simulink model "tricycle_pathstations"  (R2021a)
settings: Solver=VariableStepAuto  StartTime=0.0  StopTime=inf  RelTol=1e-3
InitFcn:
  | i=1
libraries: simulink_extras x3, vehdynlibviscommon x1
settings Model: Creator=EGYPT  LastModifiedBy=Mostafa Ali
settings SolverCC: AlgebraicLoopSolver=TrustRegion
settings DebuggingCC: SFMachineParentedDataDiag=warning

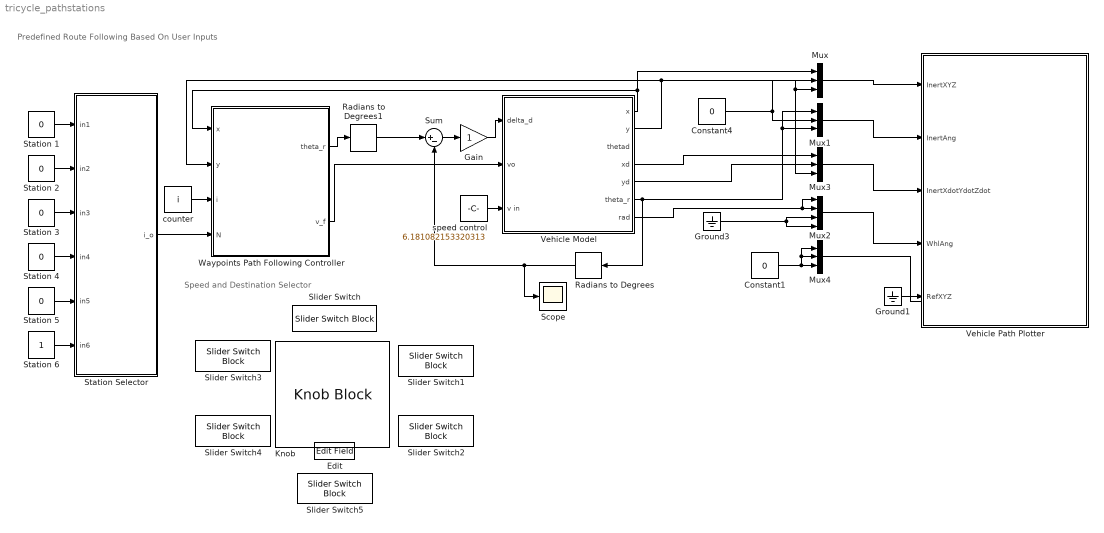
== system tricycle_pathstations ==
  note: Predefined Route Following Based On User Inputs
  note: Speed and Destination Selector
  Constant1 : Constant  Value=0
  Constant4 : Constant  Value=0
  Edit : EditField  LabelPosition=Hide  ShowInitialText=on  Alignment=Center
  Gain : Gain
  Ground1 : Ground
  Ground3 : Ground
  Knob : KnobBlock  ScaleMax=10
  Mux{,1,3..4} (4 alike) : Mux  Inputs=3
  Mux2 : Mux
  Radians to Degrees : simulink_extras/Transformations/Radians to Degrees
  Radians to Degrees1 : simulink_extras/Transformations/Radians to Degrees
  Scope : Scope
  Slider Switch{,1..5} (6 alike) : SliderSwitchBlock
      settings: Values={{'Off', 'On'}, [0 1]}
  Station {1..5} (5 alike) : Constant  Value=0
  Station 6 : Constant
  "Station Selector " : MATLAB Function  TreatAsAtomicUnit=on
  Sum : Sum  Inputs=|+-
  "Vehicle Model " : Subsystem
      mask Display: image('D:\grad 1\matlab\maskKM.JPG'); % Use "Edit Image" on toolstrip to change.
  Vehicle Path Plotter : Subsystem  mask(Vehicle XY Plotter){extRef=on, extStats=off, extTireF=off, a=2, b=2, w=2, figBorder=10, bufferSize=1024, velNorm=5, tireFNorm=1000, pltDT=0.2}
      mask prompts: extRef "Plot path reference, extRef"; extStats "Display speed, RPM and Gear"; extTireF "Display tire forces"; a "Distance to front axle from CG, a [m]:"; b "Distance to rear axle from CG, b [m]:"; w "Track width, w [m]:"; figBorder "Distance to figure borders, figBorder [m]:"; bufferSize "Path buffer sampe size, bufferSize []:"; velNorm "Velocity vector scaling, velNorm [m*s/m]:"; tireFNorm "Tire force vector scaling, tireFNorm [m/N]:"; pltDT "Plot update rate, pltDT [s]:"
      mask help:
      | This block will display a MATLAB figure which indicates the vehicle path, current position and heading velocity.
      | An optional path reference is also provided.
      mask init:
      | block = gcb;
      | if autoblkschecksimstopped(block)
      |     ParamNames = {'extRef';'extStats';'extTireF';'extTireF'};
      |     PortNames = {'RefXYZ';'Stats';'TireFx';'TireFy'};
      |     for idx=1:length(PortNames)
      |         InportOption  = {'built-in/Ground', [PortNames{idx}, ' Ground'];...
      |             'built-in/Inport',PortNames{idx}};
      |         if ~strcmp(get_param(block,ParamNames{idx}),'on')
      |             NewBlkHdl = autoblksreplaceblock(block, InportOption, 1);
      |             set_param(NewBlkHdl, 'ShowName', 'off');
      |         else
      |             autoblksreplaceblock(block, InportOption, 2);
      |         end
      |     end
      |     InportNames = {'InertXYZ';'InertAng';'InertXdotYdotZdot';'WhlAng';'RefXYZ';'Stats';'TireFx';'TireFy'};
      |     FoundNames = get_param(find_system(block, 'LookUnderMasks', 'all', 'SearchDepth', 1, 'FollowLinks', 'on', 'BlockType', 'Inport'), 'Name');
      |     [~,PortI] = intersect(InportNames, FoundNames);
      |     PortI = sort(PortI);
      |     for idx = 1:length(PortI)
      |         set_param([block, '/', InportNames{PortI(idx)}], 'Port', num2str(idx));
      |     end
      | end
      mask TypeOptions a: Vehicle XY Plotter/a
      mask TypeOptions b: Vehicle XY Plotter/b
      mask TypeOptions w: Vehicle XY Plotter/w
      mask TypeOptions figBorder: Vehicle XY Plotter/figBorder
      mask TypeOptions bufferSize: Vehicle XY Plotter/bufferSize
      mask TypeOptions velNorm: Vehicle XY Plotter/velNorm
      mask TypeOptions tireFNorm: Vehicle XY Plotter/tireFNorm
      mask DialogControl Container3 Prompt: Plot and Display Options
  "Waypoints Path Following Controller " : MATLAB Function  TreatAsAtomicUnit=on
  counter : Constant  Value=i
  speed control : Constant  Value=6.181082153320313
  wires:
  Radians to Degrees/1 -> Sum/2, Scope/1
  Mux3/1 -> Vehicle Path Plotter/3(InertXdotYdotZdot)
  "Vehicle Model "/5(yd) -> Mux3/2
  speed control/1 -> "Vehicle Model "/3(v in)
  Radians to Degrees1/1 -> Sum/1
  "Vehicle Model "/1(x) -> Mux/1, "Waypoints Path Following Controller "/1(x)
  Ground3/1 -> Mux2/3, Mux2/4
  "Waypoints Path Following Controller "/1(theta_r) -> Radians to Degrees1/1
  Mux/1 -> Vehicle Path Plotter/1(InertXYZ)
  Sum/1 -> Gain/1
  Mux1/1 -> Vehicle Path Plotter/2(InertAng)
  "Vehicle Model "/2(y) -> Mux/2, "Waypoints Path Following Controller "/2(y)
  "Vehicle Model "/4(xd) -> Mux3/1
  Constant1/1 -> Mux4/1, Mux4/2, Mux4/3
  Mux2/1 -> Vehicle Path Plotter/4(WhlAng)
  Gain/1 -> "Vehicle Model "/1(delta_d)
  Mux4/1 -> Vehicle Path Plotter/5(RefXYZ)
  Constant4/1 -> Mux3/3, Mux/3, Mux1/2
  "Vehicle Model "/6(theta_r) -> Mux1/1, Mux1/3, Radians to Degrees/1
  Station 1/1 -> "Station Selector "/1(in1)
  Station 2/1 -> "Station Selector "/2(in2)
  Station 3/1 -> "Station Selector "/3(in3)
  Station 4/1 -> "Station Selector "/4(in4)
  Station 5/1 -> "Station Selector "/5(in5)
  Station 6/1 -> "Station Selector "/6(in6)
  "Station Selector "/1(i_o) -> "Waypoints Path Following Controller "/4(N)
  counter/1 -> "Waypoints Path Following Controller "/3(i)
  "Vehicle Model "/7(rad) -> Mux2/1, Mux2/2
  Ground1/1 -> ?
  "Waypoints Path Following Controller "/2(v_f) -> "Vehicle Model "/2(vo)

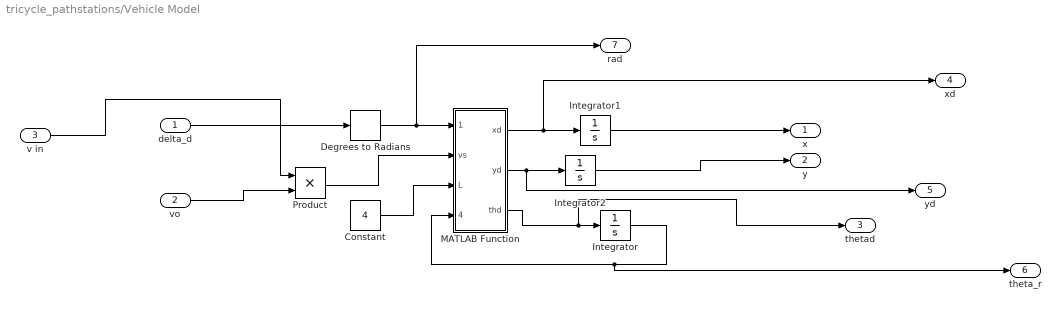
== system tricycle_pathstations/Vehicle Model  ==
  delta_d : Inport
  vo : Inport  Port=2
  v in : Inport  Port=3
  Constant : Constant  Value=4
  Degrees to Radians : simulink_extras/Transformations/Degrees to Radians
  Integrator : Integrator
  Integrator1 : Integrator
  Integrator2 : Integrator
  MATLAB Function : MATLAB Function  TreatAsAtomicUnit=on
  Product : Product
  x : Outport
  y : Outport  Port=2
  thetad : Outport  Port=3
  xd : Outport  Port=4
  yd : Outport  Port=5
  theta_r : Outport  Port=6
  rad : Outport  Port=7
  wires:
  Integrator/1 -> theta_r/1, MATLAB Function/4(theta_r)
  Degrees to Radians/1 -> rad/1, MATLAB Function/1(delta_r)
  MATLAB Function/1(xd) -> xd/1, Integrator1/1
  Integrator2/1 -> y/1
  Product/1 -> MATLAB Function/2(vs)
  MATLAB Function/3(thd) -> thetad/1, Integrator/1
  Constant/1 -> MATLAB Function/3(L)
  MATLAB Function/2(yd) -> yd/1, Integrator2/1
  v in/1 -> Product/1
  delta_d/1 -> Degrees to Radians/1
  Integrator1/1 -> x/1
  vo/1 -> Product/2

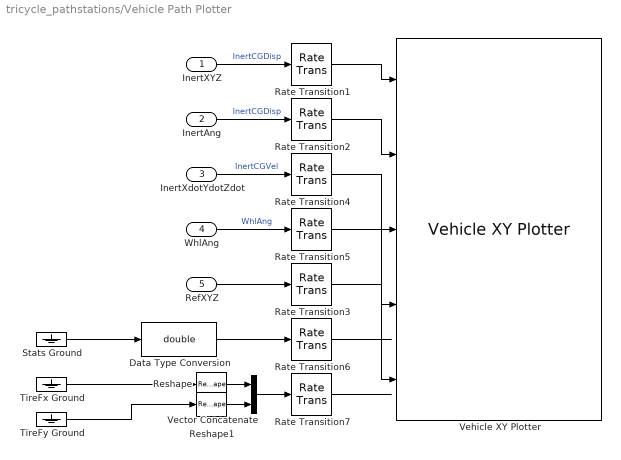
== system tricycle_pathstations/Vehicle Path Plotter ==
  InertXYZ : Inport
  InertAng : Inport  Port=2
  InertXdotYdotZdot : Inport  Port=3
  WhlAng : Inport  Port=4
  RefXYZ : Inport  Port=5
  Data Type Conversion : DataTypeConversion  OutDataTypeStr=double
  Rate Transition{1..7} (7 alike) : RateTransition  Deterministic=off  OutPortSampleTime=pltDT
  Reshape : Reshape  OutputDimensionality=Row vector (2-D)
  Reshape1 : Reshape  OutputDimensionality=Row vector (2-D)
  Stats Ground : Ground
  TireFx Ground : Ground
  TireFy Ground : Ground
  Vector Concatenate : Concatenate  Mode=Multidimensional array
  Vehicle XY Plotter : vehdynlibviscommon/Vehicle XY Plotter  w=w  a=a  b=b  figBorder=figBorder  bufferSize=bufferSize  extStats=off  extTireF=off
      settings: SourceProductBaseCode=VE
  wires:
  Vector Concatenate/1 -> Rate Transition7/1
  Reshape1/1 -> Vector Concatenate/2
  Reshape/1 -> Vector Concatenate/1
  RefXYZ/1 -> Rate Transition3/1
  Rate Transition7/1 -> ?
  Data Type Conversion/1 -> Rate Transition6/1
  Rate Transition6/1 -> ?
  Rate Transition5/1 -> Vehicle XY Plotter/4
  Rate Transition4/1 -> Vehicle XY Plotter/3
  Rate Transition2/1 -> Vehicle XY Plotter/2
  Rate Transition1/1 -> Vehicle XY Plotter/1
  Rate Transition3/1 -> Vehicle XY Plotter/5
  WhlAng/1 -> Rate Transition5/1  "WhlAng"
  InertXYZ/1 -> Rate Transition1/1  "InertCGDisp"
  InertXdotYdotZdot/1 -> Rate Transition4/1  "InertCGVel"
  InertAng/1 -> Rate Transition2/1  "InertCGDisp"
  TireFx Ground/1 -> Reshape/1
  TireFy Ground/1 -> Reshape1/1
  Stats Ground/1 -> Data Type Conversion/1

== matlab function tricycle_pathstations/Waypoints Path Following Controller  ==
  settings: updateMethod=DISCRETE
  data: x input; theta_r output; y input; v_f output; i input; N input
function [theta_r,v_f]   = fcn(x,y,i,N)
persistent i2 
if isempty(i2)
        i2=i;
end
  
xw=[0,0,0,20,20,20,0]
yw=[0,50,100,100,50,0,0]
r_min=1
xr=xw(i2)
yr=yw(i2)
dx=xr-x
dy=yr-y
q=((dx)^2)+((dy)^2)
r=sqrt(q)
theta_r=atan2(dy,dx)
if (r<r_min)
    if (i2<N)
      v_f=1;
      i2=i2+1 ;
    elseif i2>6
       v_f=1;
        i2=1;
    else
          v_f=0;
        end
    else
v_f=1  
end

== matlab function tricycle_pathstations/Vehicle Model /MATLAB Function ==
  data: delta_r input; xd output; yd output; thd output; vs input; L input; theta_r input
function[xd,yd,thd] = fcn(delta_r,vs,L,theta_r)
xd=vs*cos(delta_r)*cos(theta_r)
yd=vs*cos(delta_r)*sin(theta_r)
thd=(vs/L)*sin(delta_r)

== matlab function tricycle_pathstations/Station Selector  ==
  data: i_o output; in1 input; in2 input; in3 input; in4 input; in5 input; in6 input
function i_o = fcn(in1, in2, in3, in4, in5,in6)
i_o=1
if (in1==1)
    i_o=2
elseif (in2==1)
    i_o=3
elseif (in3==1)
    i_o=4
elseif (in4==1)
    i_o=5
elseif (in5==1)
    i_o=6
elseif (in6==1)
    i_o=7
end
